simulink model "q_velocity_control"  (R2018b)
settings: Solver=ode1  StartTime=0.0  StopTime=20  FixedStep=0.002  RelTol=1e-3  EnableMultiTasking=on
undefined symbols (not defined in the file or in its folder): HIL, qc_get_step_size
libraries: quarc_library x4, simulink x1
settings Model: SimulationMode=external  ExtModeTrigDuration=10000  Creator=Control_Eng  LastModifiedBy=Student
settings SolverCC: PositivePriorityOrder=on
settings DataIOCC: LimitDataPoints=on  SaveFormat=Array
settings OptimizationCC: LifeSpan=inf
settings DebuggingCC: SolverPrmCheckMsg=warning  SFUnexpectedBacktrackingDiag=warning  SFNoUnconditionalDefaultTransitionDiag=warning  SFExecutionAtInitializationDiag=none
settings HardwareCC: ProdBitPerPointer=32  ProdBitPerSizeT=32  ProdBitPerPtrDiffT=32  ProdLargestAtomicFloat=None  ProdIntDivRoundTo=Undefined  ProdEndianess=Unspecified  ProdWordSize=32  ProdHWDeviceType=32-bit Generic
settings ModelReferenceCC: PropagateSignalLabelsOutOfModel=off
settings SFSimCC: SimUseLocalCustomCode=off
settings RTWCC: SystemTargetFile=quarc_win64.tlc  TemplateMakefile=quarc_default_tmf  Description=QUARC Win64 Target  RTWUseLocalCustomCode=off
settings CodeAppCC: StateflowObjectComments=on
settings STFCustomTargetCC: TargetPreCompLibLocation=C:\PROGRA~3\QUARC\lib\2014a\win64\release  ConcurrentExecutionCompliant=on  GeneratePreprocessorConditionals=Disable all  CombineOutputUpdateFcns=on  SystemTargetFile=quarc_win64.tlc
settings GRTTargetCC: TargetPreCompLibLocation=C:\PROGRA~3\QUARC\lib\2018b\win64\release  TargetLangStandard=C89/C90 (ANSI)  ParMdlRefBuildCompliant=off  CompOptLevelCompliant=off  GeneratePreprocessorConditionals=Disable all  MatFileLogging=off  CPPClassGenCompliant=off  UseToolchainInfoCompliant=off  ExtMode=on  ExtModeMexFile=quarc_comm
settings ConfigComp: CovMetricSettings=dw  CovHtmlReporting=on  CovSaveCumulativeToWorkspaceVar=on  CovSaveSingleToWorkspaceVar=on  CovExternalEMLEnable=off  CovSFcnEnable=off

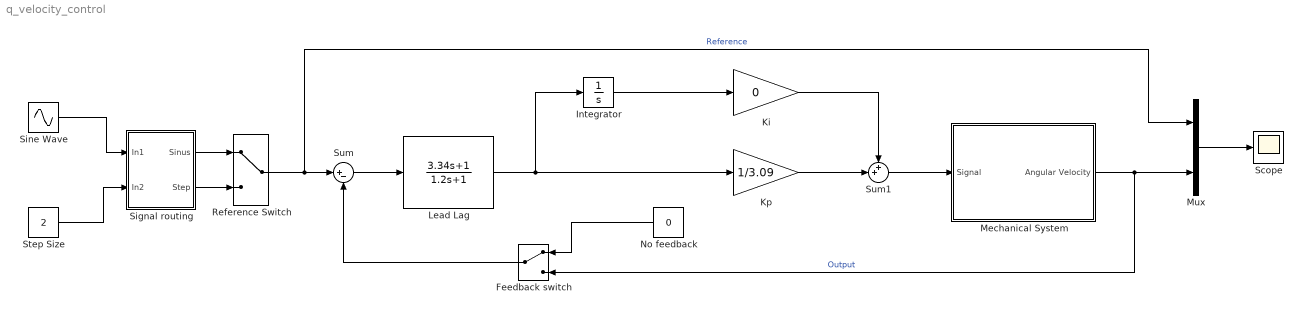
== system q_velocity_control ==
  Feedback switch : ManualSwitch
  Integrator : Integrator
  Ki : Gain  Gain=0
  Kp : Gain  Gain=1/3.09
  Lead Lag : TransferFcn  Numerator=[3.34, 1]  Denominator=[1.2, 1]
  Mechanical System : Subsystem
  Mux : Mux  Inputs=2
  No feedback : Constant  Value=0
  Reference Switch : ManualSwitch
  Scope : Scope
  Signal routing : Subsystem
  Sine Wave : Sin  Amplitude=0.5  Bias=2  Phase=-2*1  SampleTime=0
  Step Size : Constant  Value=2
  Sum : Sum  Inputs=|+-
  Sum1 : Sum  Inputs=++|
  wires:
  Sum/1 -> Lead Lag/1
  Integrator/1 -> Ki/1
  Ki/1 -> Sum1/1
  Reference Switch/1 -> Mux/1, Sum/1  "Reference"
  Mux/1 -> Scope/1
  Kp/1 -> Sum1/2
  Lead Lag/1 -> Kp/1, Integrator/1
  Sum1/1 -> Mechanical System/1(Signal)
  Feedback switch/1 -> Sum/2
  Mechanical System/1(Angular Velocity) -> Feedback switch/2, Mux/2  "Output"
  No feedback/1 -> Feedback switch/1
  Sine Wave/1 -> Signal routing/1(In1)
  Step Size/1 -> Signal routing/2(In2)
  Signal routing/1(Sinus) -> Reference Switch/1
  Signal routing/2(Step) -> Reference Switch/2

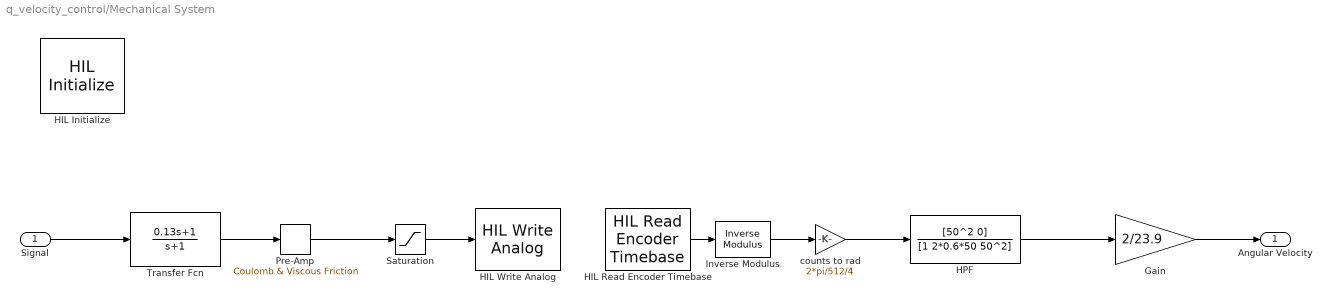
== system q_velocity_control/Mechanical System ==
  Signal : Inport
  Gain : Gain  Gain=2/23.9
  HIL Initialize : quarc_library/Data Acquisition/Generic/Configuration/HIL Initialize  Priority=-99  object_name=HIL-1  board_type=qube_servo_usb  board_number=0  board_options=d0=pwm;d1=pwm;led=auto;update_rate=normal;decimation=1  exclusive=off  active=off  hardware_clocks=[0]  clock_modes=[]  initial_clock_frequencies=[]  set_clock_params_at_start=off  set_clock_params_at_switch_in=off  set_clock_frequencies_at_start=off  set_clock_frequencies_at_switch_in=off  analog_input_channels=[]  analog_input_configurations=[]  analog_input_maximums=[]  analog_input_minimums=[]  set_analog_input_params_at_start=off  set_analog_input_params_at_switch_in=off  analog_output_channels=[0:1]  analog_output_maximums=10  analog_output_minimums=-10  initial_analog_outputs=[0]  final_analog_outputs=[0]  watchdog_analog_outputs=0  set_analog_output_params_at_start=on  set_analog_output_params_at_switch_in=off  set_analog_outputs_at_start=on  set_analog_outputs_at_switch_in=off  set_analog_outputs_at_terminate=on  set_analog_outputs_at_switch_out=off  set_analog_outputs_on_watchdog=off  digital_input_channels=[]  digital_output_channels=[]  digital_output_configuration=[]  initial_digital_outputs=[]  final_digital_outputs=[]  watchdog_digital_outputs=[]  set_digital_output_params_at_start=off  set_digital_output_params_at_switch_in=off  set_digital_outputs_at_start=off  set_digital_outputs_at_switch_in=off  set_digital_outputs_at_terminate=off  set_digital_outputs_at_switch_out=off  set_digital_outputs_on_watchdog=off  encoder_channels=[0:1]  quadrature=[4]  encoder_filter_frequency=[]  initial_encoder_counts=[0]  set_encoder_params_at_start=on  set_encoder_params_at_switch_in=off  set_encoder_counts_at_start=on  set_encoder_counts_at_switch_in=off  pwm_channels=[]  pwm_modes=[]  pwm_frequency=[]  pwm_configuration=[]  pwm_alignment=[]  pwm_polarity=[]  pwm_leading_deadband=[]  pwm_trailing_deadband=[]  initial_pwm_outputs=[]  final_pwm_outputs=[]  watchdog_pwm_outputs=[]  set_pwm_params_at_start=off  set_pwm_params_at_switch_in=off  set_pwm_outputs_at_start=off  set_pwm_outputs_at_switch_in=off  set_pwm_outputs_at_terminate=off  set_pwm_outputs_at_switch_out=off  set_pwm_outputs_on_watchdog=off  other_output_channels=[]  initial_other_outputs=[]  final_other_outputs=[]  watchdog_other_outputs=[]  set_other_outputs_at_start=off  set_other_outputs_at_switch_in=off  set_other_outputs_at_terminate=off  set_other_outputs_at_switch_out=off  set_other_outputs_on_watchdog=off
  HIL Read Encoder Timebase : quarc_library/Data Acquisition/Generic/Timebases/HIL Read Encoder Timebase  object_name=HIL-1  clock=0  channels=0  samples_in_buffer=max(ceil(1/qc_get_step_size), 1)  active=on  vector_output=off  data_type_mode=Inherit via back propagation  data_type=double
  HIL Write Analog : quarc_library/Data Acquisition/Generic/Immediate I//O/HIL Write Analog  object_name=HIL-1  channels=[0]  sample_time=-1  active=off  vector_input=off
  HPF : TransferFcn  Numerator=[50^2 0]  Denominator=[1 2*0.6*50 50^2]
  Inverse Modulus : quarc_library/Discontinuities/Inverse Modulus  modulus=2^16  output_derivative=off  output_revolutions=off  max_x=Inf  min_x=-Inf
  Pre-Amp : simulink/Discontinuities/Coulomb & Viscous Friction  offset=pre_amp  gain=1
      settings: SourceProductName=Simulink
  Saturation : Saturate  UpperLimit=10  LowerLimit=-10
  Transfer Fcn : TransferFcn  Numerator=[0.13 1]  Denominator=[1 1]
  counts to rad : Gain  Gain=2*pi/512/4
  Angular Velocity : Outport
  wires:
  HIL Read Encoder Timebase/1 -> Inverse Modulus/1
  Signal/1 -> Transfer Fcn/1
  Gain/1 -> Angular Velocity/1
  Transfer Fcn/1 -> Pre-Amp/1
  Inverse Modulus/1 -> counts to rad/1
  Saturation/1 -> HIL Write Analog/1
  Pre-Amp/1 -> Saturation/1
  counts to rad/1 -> HPF/1
  HPF/1 -> Gain/1

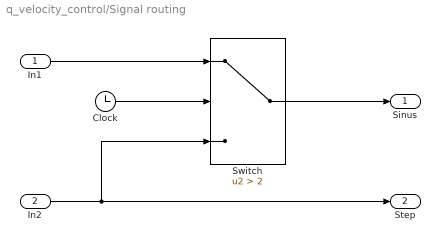
== system q_velocity_control/Signal routing ==
  In1 : Inport
  In2 : Inport  Port=2
  Clock : Clock
  Switch : Switch  Criteria=u2 > Threshold  Threshold=2
  Sinus : Outport
  Step : Outport  Port=2
  wires:
  Clock/1 -> Switch/2
  In2/1 -> Step/1, Switch/3
  In1/1 -> Switch/1
  Switch/1 -> Sinus/1
